simulink model "FUNCTIONING_SC"  (R2022b)
settings: Solver=FixedStepAuto  StartTime=0.0  StopTime=10.0  FixedStep=1e-3  RelTol=1e-3  EnableMultiTasking=on
undefined symbols (not defined in the file): D0, D1, D10, D11, D12, D13, D2, D3, D4, D5, D6, D7, D8, D9, PTA0, PTA1, PTA2, PTB23, PTB9, PTC16, PTC17, PTC2, PTC3, PTC4, PTD0, PTD1, PTD2, PTD3
libraries: frdmk64flib x19, etargetslib x3
settings Model: ExtModeTrigDuration=5  Creator=Hakam  LastModifiedBy=Hakam
settings OptimizationCC: EnhancedBackFolding=on  PassReuseOutputArgsAs=Individual arguments  ZeroExternalMemoryAtStartup=off  ZeroInternalMemoryAtStartup=off  MaxStackSize=64  OptimizeBlockOrder=speed  DifferentSizesBufferReuse=on  OptimizationCustomize=off  EfficientTunableParamExpr=on
settings DebuggingCC: ParameterTunabilityLossMsg=error
settings HardwareCC: ProdBitPerPointer=32  ProdBitPerSizeT=32  ProdBitPerPtrDiffT=32  ProdLargestAtomicInteger=Long  ProdLargestAtomicFloat=Double  ProdWordSize=32  ProdHWDeviceType=ARM Compatible->ARM Cortex
settings SFSimCC: MATLABDynamicMemAlloc=off
settings RTWCC: Description=Embedded Coder  SystemTargetFile=ert.tlc  HardwareBoard=NXP FRDM-K64F  TLCOptions="-aInlineSetEventsForThisBaseRateFcn=TLC_FALSE -aSuppressMultiTaskScheduler=TLC_FALSE  -aRateBasedStepFcn=0"  TemplateMakefile=ert_default_tmf  Toolchain=GNU Tools for ARM Embedded Processors
settings CodeAppCC: ForceParamTrailComments=on  IgnoreCustomStorageClasses=off  OperatorAnnotations=on  SimulinkDataObjDesc=on  SFDataObjDesc=on  InsertBlockDesc=on
settings ERTTargetCC: ExtModeTransport=4  ExtModeMexFile=sendToCommService

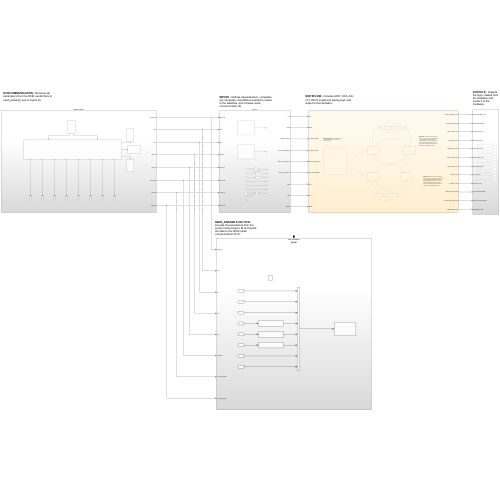
[thumbnail: Simulink's stored preview of the top-level diagram]
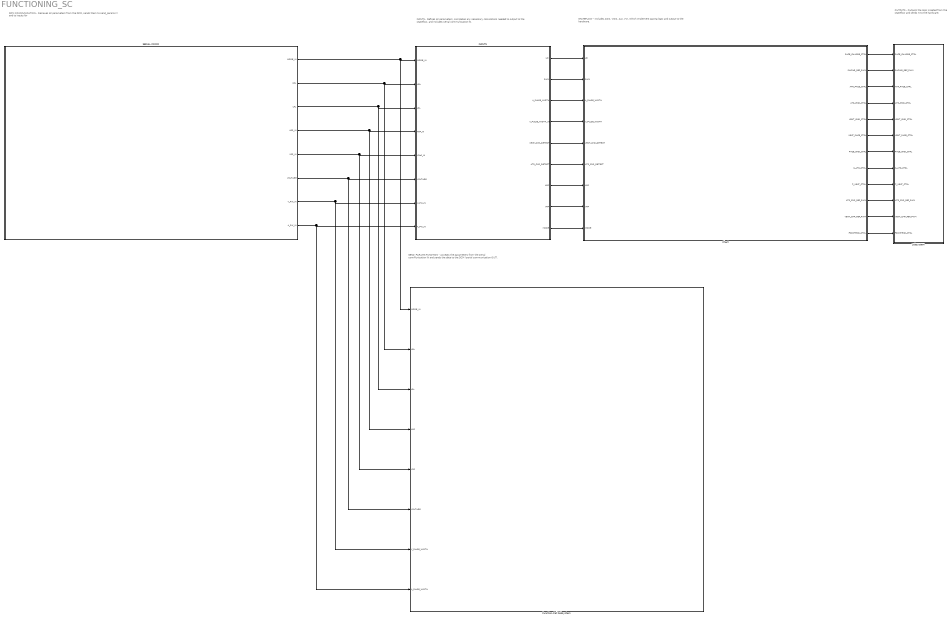
== system FUNCTIONING_SC ==
  note: INPUTS - Defines all parameters, completes any necessary calculations needed to output to the stateflow, and includes serial communication IN.
  note: STATEFLOW - Includes AOO, VOO, AAI, VVI, Which implement pacing logic and output to the hardware.
  note: SEND_PARAMS FUNCTION - Accepts the parameters from the serial communication IN and sends the data to the DCM (serial communication OUT).
  note: OUTPUTS - Outputs the logic created from the stateflow and sends it to the hardware.
  note: DCM COMMUNICATION - Recieves all parameters from the DCM, sends them to send_params() and to inputs for
  Chart : Stateflow chart  TreatAsAtomicUnit=on
      settings: PortSchema="{\"entries\":[{\"content\":{\"sides\":[{\"content\":{\"connectorIds\":[\"In5\",\"In2\",\"In1\",\"In7\",\"In3\",\"In4\",\"In6\",\"In9\",\"In8\"]},\"type\":\"ConnectorPlacement.EquallySpacedRectSide\",\"uuid\":\"579a0715-eecf-4ad1-b9c7-876da5a2f487\"},{\"content\":{\"connectorIds\":[\"Out1\",\"Out2\",\"Out3\",\"Out4\",\"Out5\",\"Out6\",\"Out7\",\"Out8\",\"Out9\",\"Out10\",\"Out11\",\"Out12\"],\"side\":\"RIGHT\"},\"type\":\"ConnectorPlacement.EquallySpacedRectSide\",\"uuid\":\"7723b8dd-9321-4ba0-a105-5fe980f58500\"},{\"content\":{\"connectorIds\":[],\"side\":\"TOP\"},\"type\":\"ConnectorPlacement.EquallySpacedRectSide\",\"uuid\":\"a2cc372f-b65a-4c95-aa24-637f5fae7d8b\"}]},\"type\":\"ConnectorPlacement.EquallySpacedConnector\",\"uuid\":\"f3293a12-0736-4187-8ed2-302834bf53da\"}],\"packageUris\":[\"http://schema.mathworks.com/mf0/Connector/R2020b\"],\"version\":\"1.0\"}"
  Function-Call Subsystem : Subsystem  TreatAsAtomicUnit=on
  INPUTS : Subsystem
      settings: PortSchema="{\"entries\":[{\"content\":{\"sides\":[{\"content\":{\"connectorIds\":[]},\"type\":\"ConnectorPlacement.EquallySpacedRectSide\",\"uuid\":\"bedbe6ad-1dc2-4cce-9585-188ab1dfdae5\"},{\"content\":{\"connectorIds\":[],\"side\":\"RIGHT\"},\"type\":\"ConnectorPlacement.EquallySpacedRectSide\",\"uuid\":\"0b0c00e6-e38b-4dbd-945a-73b1885ed563\"},{\"content\":{\"connectorIds\":[\"In1\",\"In2\",\"In3\",\"In4\",\"In5\",\"In6\",\"In7\",\"In8\"],\"side\":\"TOP\"},\"type\":\"ConnectorPlacement.EquallySpacedRectSide\",\"uuid\":\"0c1f6ce2-499b-446e-a336-8c6519be34d0\"},{\"content\":{\"connectorIds\":[\"Out1\",\"Out2\",\"Out3\",\"Out4\",\"Out5\",\"Out6\",\"Out7\",\"Out8\",\"Out9\"],\"side\":\"BOTTOM\"},\"type\":\"ConnectorPlacement.EquallySpacedRectSide\",\"uuid\":\"510989f2-1dca-4772-b500-383bd8bd4f04\"}]},\"type\":\"ConnectorPlacement.EquallySpacedConnector\",\"uuid\":\"2b867d07-0d3f-4ca3-b154-a8d01fc9a05c\"}],\"packageUris\":[\"http://schema.mathworks.com/mf0/Connector/R2020b\"],\"version\":\"1.0\"}"
  SERIAL COMM : Subsystem
      settings: PortSchema="{\"entries\":[{\"content\":{\"sides\":[{\"content\":{\"connectorIds\":[]},\"type\":\"ConnectorPlacement.EquallySpacedRectSide\",\"uuid\":\"bedbe6ad-1dc2-4cce-9585-188ab1dfdae5\"},{\"content\":{\"connectorIds\":[],\"side\":\"RIGHT\"},\"type\":\"ConnectorPlacement.EquallySpacedRectSide\",\"uuid\":\"0b0c00e6-e38b-4dbd-945a-73b1885ed563\"},{\"content\":{\"connectorIds\":[],\"side\":\"TOP\"},\"type\":\"ConnectorPlacement.EquallySpacedRectSide\",\"uuid\":\"0c1f6ce2-499b-446e-a336-8c6519be34d0\"},{\"content\":{\"connectorIds\":[\"Out1\",\"Out2\",\"Out3\",\"Out4\",\"Out5\",\"Out6\",\"Out7\",\"Out8\"],\"side\":\"BOTTOM\"},\"type\":\"ConnectorPlacement.EquallySpacedRectSide\",\"uuid\":\"510989f2-1dca-4772-b500-383bd8bd4f04\"}]},\"type\":\"ConnectorPlacement.EquallySpacedConnector\",\"uuid\":\"2b867d07-0d3f-4ca3-b154-a8d01fc9a05c\"}],\"packageUris\":[\"http://schema.mathworks.com/mf0/Connector/R2020b\"],\"version\":\"1.0\"}"
  Subsystem : Subsystem
  wires:
  SERIAL COMM/4(ARP_IN) -> Function-Call Subsystem/4(ARP), INPUTS/4(ARP_IN)
  INPUTS/6(ATR_CMP_DETECT) -> Chart/4(ATR_CMP_DETECT)
  INPUTS/2(PWM) -> Chart/2(PWM)
  INPUTS/7(ARP) -> Chart/6(ARP)
  Chart/6(VENT_PACE_CTRL) -> Subsystem/6(VENT_PACE_CTRL)
  INPUTS/9(MODE) -> Chart/8(MODE)
  INPUTS/4(V_PULSE_WIDTH_IN) -> Chart/7(V_PULSE_WIDTH)
  SERIAL COMM/7(V_PW_IN) -> INPUTS/7(V_PW_IN), Function-Call Subsystem/7(V_PULSE_WIDTH)
  INPUTS/8(VRP) -> Chart/9(VRP)
  Chart/3(ATR_PACE_CTRL) -> Subsystem/3(ATR_PACE_CTRL)
  Chart/8(Z_ATR_CTRL) -> Subsystem/8(Z_ATR_CTRL)
  Chart/9(Z_VENT_CTRL) -> Subsystem/9(Z_VENT_CTRL)
  SERIAL COMM/5(VRP_IN) -> Function-Call Subsystem/5(VRP), INPUTS/5(VRsP_IN)
  SERIAL COMM/1(MODE_IN) -> Function-Call Subsystem/1(MODE_IN), INPUTS/1(MODE_IN)
  Chart/10(ATR_CMP_REF_PWM) -> Subsystem/10(ATR_CMP_REF_PWM)
  Chart/5(VENT_GND_CTRL) -> Subsystem/5(VENT_GND_CTRL)
  Chart/12(FRONTEND_CTRL) -> Subsystem/12(FRONTEND_CTRL)
  Chart/4(ATR_GND_CTRL) -> Subsystem/4(ATR_GND_CTRL)
  Chart/7(PACE_GND_CTRL) -> Subsystem/7(PACE_GND_CTRL)
  Chart/11(VENT_CMP_REF_PWM) -> Subsystem/11(VENT_CMP_REF_PWM)
  Chart/1(PACE_CHARGE_CTRL) -> Subsystem/1(PACE_CHARGE_CTRL)
  SERIAL COMM/6(VOLTAGE) -> Function-Call Subsystem/6(VOLTAGE), INPUTS/6(VOLTAGE)
  Chart/2(PACING_REF_PWM) -> Subsystem/2(PACING_REF_PWM)
  INPUTS/5(VENT_CMP_DETECT) -> Chart/3(VENT_CMP_DETECT)
  SERIAL COMM/3(LRL) -> INPUTS/3(LRL), Function-Call Subsystem/3(LRL)
  INPUTS/1(LRI) -> Chart/5(LRI)
  INPUTS/3(A_PULSE_WIDTH) -> Chart/1(A_PULSE_WIDTH)
  SERIAL COMM/2(URL) -> INPUTS/2(URL), Function-Call Subsystem/2(URL)
  SERIAL COMM/8(A_PW_IN) -> INPUTS/8(A_PW_IN), Function-Call Subsystem/8(A_PULSE_WIDTH)

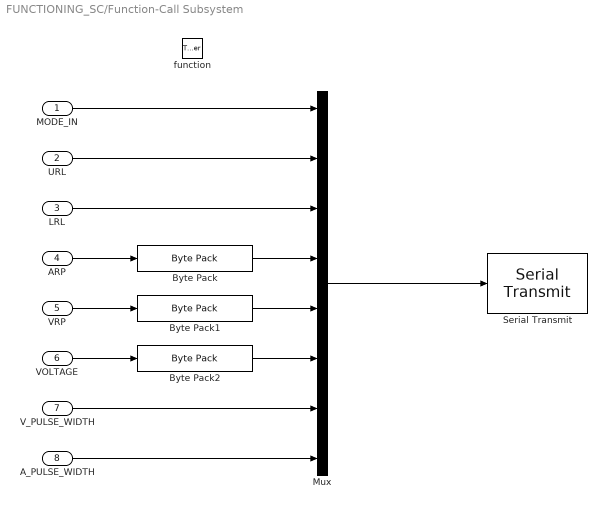
== system FUNCTIONING_SC/Function-Call Subsystem ==
  MODE_IN : Inport
  URL : Inport  Port=2
  LRL : Inport  Port=3
  ARP : Inport  Port=4
  VRP : Inport  Port=5
  VOLTAGE : Inport  Port=6  OutDataTypeStr=single
  V_PULSE_WIDTH : Inport  Port=7
  A_PULSE_WIDTH : Inport  Port=8
  function : TriggerPort  TriggerType=function-call  IsSimulinkFunction=on  FunctionName=send_parameters  VariantControl=(inherit)
  Byte Pack : etargetslib/Byte Pack  datatypes={'uint16'}  byteAlign=1
  Byte Pack1 : etargetslib/Byte Pack  datatypes={'uint16'}  byteAlign=1
  Byte Pack2 : etargetslib/Byte Pack  datatypes={'single'}  byteAlign=1
  Mux : Mux  Inputs=8
  Serial Transmit : frdmk64flib/Serial Transmit  SCIModule=0  Baudrate=uint32(9600)  Parity=None  StopBits=1  HardwareFlowControl=None  ByteOrder=LittleEndian  BlockingMode=on  OutputStatus=off
  wires:
  Mux/1 -> Serial Transmit/1
  A_PULSE_WIDTH/1 -> Mux/8
  Byte Pack/1 -> Mux/4
  ARP/1 -> Byte Pack/1
  VRP/1 -> Byte Pack1/1
  Byte Pack1/1 -> Mux/5
  V_PULSE_WIDTH/1 -> Mux/7
  MODE_IN/1 -> Mux/1
  LRL/1 -> Mux/3
  URL/1 -> Mux/2
  Byte Pack2/1 -> Mux/6
  VOLTAGE/1 -> Byte Pack2/1

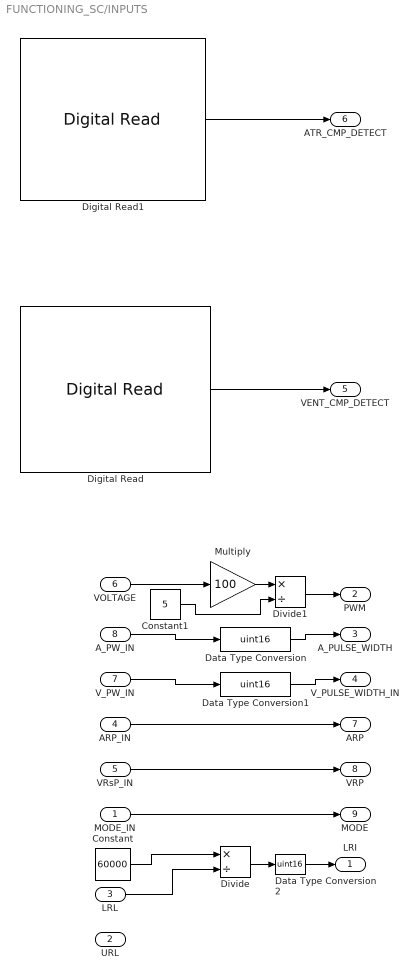
== system FUNCTIONING_SC/INPUTS ==
  MODE_IN : Inport
  URL : Inport  Port=2
  LRL : Inport  Port=3
  ARP_IN : Inport  Port=4
  VRsP_IN : Inport  Port=5
  VOLTAGE : Inport  Port=6
  V_PW_IN : Inport  Port=7
  A_PW_IN : Inport  Port=8
  Constant : Constant  Value=60000
  Constant1 : Constant  Value=5
  Data Type Conversion : DataTypeConversion  OutDataTypeStr=uint16  SaturateOnIntegerOverflow=off  RndMeth=Floor
  Data Type Conversion1 : DataTypeConversion  OutDataTypeStr=uint16  SaturateOnIntegerOverflow=off  RndMeth=Floor
  Data Type Conversion2 : DataTypeConversion  OutDataTypeStr=uint16  SaturateOnIntegerOverflow=off  RndMeth=Floor
  Digital Read : frdmk64flib/Digital Read  Whichpin=PTC17 (D1)  SampleTime=-1
  Digital Read1 : frdmk64flib/Digital Read  Whichpin=PTC16 (D0)  SampleTime=-1
  Divide : Product  Inputs=*/
  Divide1 : Product  Inputs=*/
  Multiply : Gain  Gain=100
  LRI : Outport
  PWM : Outport  Port=2
  A_PULSE_WIDTH : Outport  Port=3
  V_PULSE_WIDTH_IN : Outport  Port=4
  VENT_CMP_DETECT : Outport  Port=5
  ATR_CMP_DETECT : Outport  Port=6
  ARP : Outport  Port=7
  VRP : Outport  Port=8
  MODE : Outport  Port=9
  wires:
  Digital Read1/1 -> ATR_CMP_DETECT/1
  Digital Read/1 -> VENT_CMP_DETECT/1
  LRL/1 -> Divide/2
  Divide/1 -> Data Type Conversion2/1
  Constant1/1 -> Divide1/2
  Multiply/1 -> Divide1/1
  Divide1/1 -> PWM/1
  Data Type Conversion/1 -> A_PULSE_WIDTH/1
  Data Type Conversion1/1 -> V_PULSE_WIDTH_IN/1
  ARP_IN/1 -> ARP/1
  VRsP_IN/1 -> VRP/1
  MODE_IN/1 -> MODE/1
  Constant/1 -> Divide/1
  A_PW_IN/1 -> Data Type Conversion/1
  Data Type Conversion2/1 -> LRI/1
  VOLTAGE/1 -> Multiply/1
  V_PW_IN/1 -> Data Type Conversion1/1

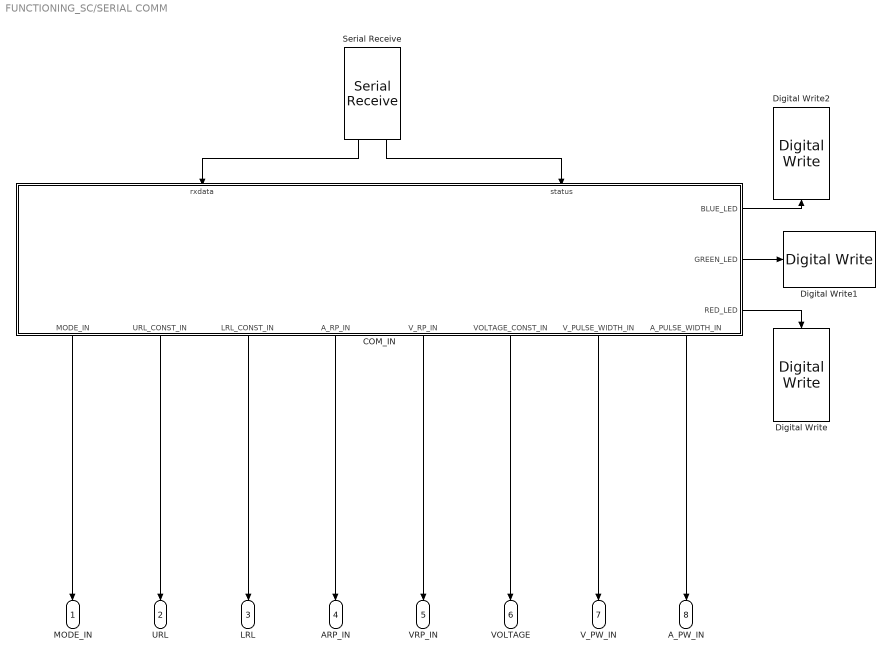
== system FUNCTIONING_SC/SERIAL COMM ==
  COM_IN : Stateflow chart  TreatAsAtomicUnit=on
      settings: PortSchema="{\"entries\":[{\"content\":{\"sides\":[{\"content\":{\"connectorIds\":[\"In1\",\"In2\"]},\"type\":\"ConnectorPlacement.EquallySpacedRectSide\",\"uuid\":\"d63df865-b51f-43d6-a13f-6ae075812ede\"},{\"content\":{\"connectorIds\":[\"Out6\",\"Out9\",\"Out4\",\"Out5\",\"Out8\",\"Out3\",\"Out7\",\"Out2\"],\"side\":\"RIGHT\"},\"type\":\"ConnectorPlacement.EquallySpacedRectSide\",\"uuid\":\"8033d1cf-b8ff-4fd5-8be7-20697f5f926f\"},{\"content\":{\"connectorIds\":[],\"side\":\"TOP\"},\"type\":\"ConnectorPlacement.EquallySpacedRectSide\",\"uuid\":\"dd3d3828-7779-4157-9ae9-dc8022e14938\"},{\"content\":{\"connectorIds\":[\"Out1\",\"Out11\",\"Out10\"],\"side\":\"BOTTOM\"},\"type\":\"ConnectorPlacement.EquallySpacedRectSide\",\"uuid\":\"0a7ca57a-2a94-44e2-b41b-d07737135386\"}]},\"type\":\"ConnectorPlacement.EquallySpacedConnector\",\"uuid\":\"07d8ed07-1da2-4ca8-9f50-15ba3dce33e0\"}],\"packageUris\":[\"http://schema.mathworks.com/mf0/Connector/R2020b\"],\"version\":\"1.0\"}"
  Digital Write : frdmk64flib/Digital Write  Whichpin=RED_LED
  Digital Write1 : frdmk64flib/Digital Write  Whichpin=GREEN_LED
  Digital Write2 : frdmk64flib/Digital Write  Whichpin=BLUE_LED
  Serial Receive : frdmk64flib/Serial Receive  SCIModule=0  Baudrate=uint32(9600)  Parity=None  StopBits=1  HardwareFlowControl=None  ByteOrder=LittleEndian  DataType=uint8  DataLength=15  BlockingMode=off  OutputStatus=on  SampleTime=-1
  MODE_IN : Outport
  URL : Outport  Port=2
  LRL : Outport  Port=3
  ARP_IN : Outport  Port=4
  VRP_IN : Outport  Port=5
  VOLTAGE : Outport  Port=6  OutDataTypeStr=single
  V_PW_IN : Outport  Port=7
  A_PW_IN : Outport  Port=8
  wires:
  COM_IN/3(VOLTAGE_CONST_IN) -> VOLTAGE/1
  Serial Receive/2 -> COM_IN/2(status)
  Serial Receive/1 -> COM_IN/1(rxdata)
  COM_IN/2(A_PULSE_WIDTH_IN) -> A_PW_IN/1
  COM_IN/5(A_RP_IN) -> ARP_IN/1
  COM_IN/6(MODE_IN) -> MODE_IN/1
  COM_IN/7(V_PULSE_WIDTH_IN) -> V_PW_IN/1
  COM_IN/8(V_RP_IN) -> VRP_IN/1
  COM_IN/4(LRL_CONST_IN) -> LRL/1
  COM_IN/9(URL_CONST_IN) -> URL/1
  COM_IN/10(RED_LED) -> Digital Write/1
  COM_IN/11(GREEN_LED) -> Digital Write1/1
  COM_IN/1(BLUE_LED) -> Digital Write2/1

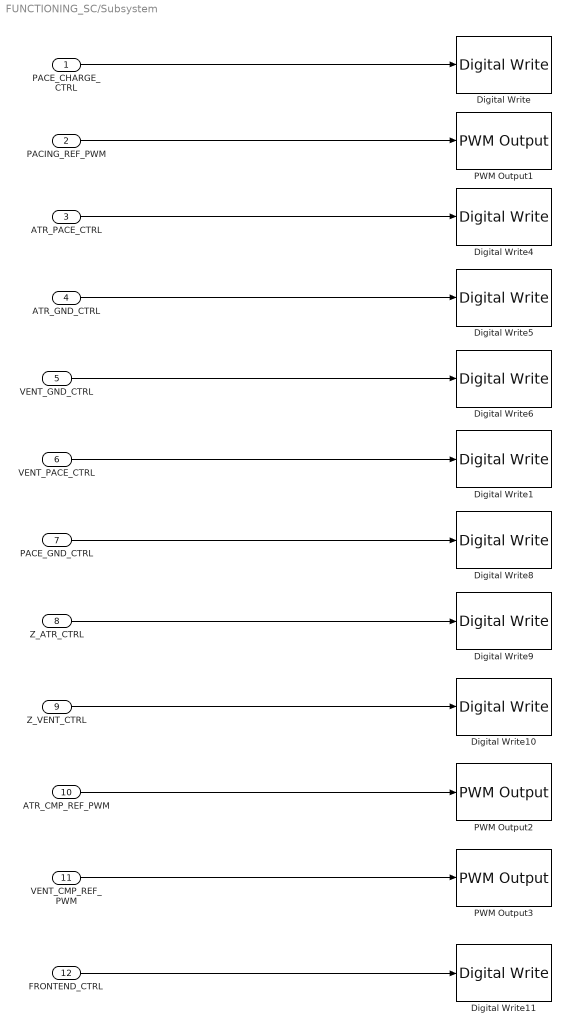
== system FUNCTIONING_SC/Subsystem ==
  PACE_CHARGE_CTRL : Inport
  PACING_REF_PWM : Inport  Port=2
  ATR_PACE_CTRL : Inport  Port=3
  ATR_GND_CTRL : Inport  Port=4
  VENT_GND_CTRL : Inport  Port=5
  VENT_PACE_CTRL : Inport  Port=6
  PACE_GND_CTRL : Inport  Port=7
  Z_ATR_CTRL : Inport  Port=8
  Z_VENT_CTRL : Inport  Port=9
  ATR_CMP_REF_PWM : Inport  Port=10
  VENT_CMP_REF_PWM : Inport  Port=11
  FRONTEND_CTRL : Inport  Port=12
  Digital Write : frdmk64flib/Digital Write  Whichpin=PTB9 (D2)
  Digital Write1 : frdmk64flib/Digital Write  Whichpin=PTC4 (D9)
  Digital Write10 : frdmk64flib/Digital Write  Whichpin=PTC3 (D7)
  Digital Write11 : frdmk64flib/Digital Write  Whichpin=PTD1 (D13)
  Digital Write4 : frdmk64flib/Digital Write  Whichpin=PTA0 (D8)
  Digital Write5 : frdmk64flib/Digital Write  Whichpin=PTD2 (D11)
  Digital Write6 : frdmk64flib/Digital Write  Whichpin=PTD3 (D12)
  Digital Write8 : frdmk64flib/Digital Write  Whichpin=PTD0 (D10)
  Digital Write9 : frdmk64flib/Digital Write  Whichpin=PTB23 (D4)
  PWM Output1 : frdmk64flib/PWM Output  Whichpin=PTA2 (D5)  InitialFrequency=2000  InitialDutyCycle=100
  PWM Output2 : frdmk64flib/PWM Output  Whichpin=PTC2 (D6)  InitialFrequency=2000  InitialDutyCycle=0
  PWM Output3 : frdmk64flib/PWM Output  Whichpin=PTA1 (D3)  InitialFrequency=2000  InitialDutyCycle=0
  wires:
  PACE_CHARGE_CTRL/1 -> Digital Write/1
  PACING_REF_PWM/1 -> PWM Output1/1
  ATR_PACE_CTRL/1 -> Digital Write4/1
  ATR_GND_CTRL/1 -> Digital Write5/1
  VENT_GND_CTRL/1 -> Digital Write6/1
  VENT_PACE_CTRL/1 -> Digital Write1/1
  PACE_GND_CTRL/1 -> Digital Write8/1
  Z_ATR_CTRL/1 -> Digital Write9/1
  Z_VENT_CTRL/1 -> Digital Write10/1
  VENT_CMP_REF_PWM/1 -> PWM Output3/1
  ATR_CMP_REF_PWM/1 -> PWM Output2/1
  FRONTEND_CTRL/1 -> Digital Write11/1

== stateflow chart FUNCTIONING_SC/SERIAL COMM/COM_IN ==
  state SET_PARAM
    entry:
    MODE_IN = rxdata(3); %Pacing modes (1-4)
    URL_CONST_IN = rxdata(4); %Upper rate limit (ppm)
    LRL_CONST_IN = rxdata(5); %Lower rate limit (ppm)
    A_RP_IN = typecast(rxdata(6:7), 'uint16'); %Refractory period (ms)
    V_RP_IN = typecast(rxdata(8:9), 'uint16'); %Refractory period (ms)
    VOLTAGE_CONST_IN =  typecast(rxdata(10:13), 'single'); %Pulse Amplitude (V)
    V_PULSE_WIDTH_IN = rxdata(14); %Pulse width (ms)
    A_PULSE_WIDTH_IN = rxdata(15); %Pulse width (ms)
    GREEN_LED=1;
    BLUE_LED = 0;
    RED_LED = 0;
  state INITIAL
    entry:
    A_PULSE_WIDTH_IN = 1;
    V_PULSE_WIDTH_IN = 2;
    VOLTAGE_CONST_IN = 1;
    LRL_CONST_IN = 1;
    A_RP_IN = 1;
    V_RP_IN = 1;
    MODE_IN = 3;
  state STANDBY
    entry:
    RED_LED=1;
    BLUE_LED = 0;
    GREEN_LED=0;
  state ECHO_PARAM
    entry:
    RED_LED = 0;
    BLUE_LED = 1;
    send_parameters();
  SET_PARAM -> STANDBY : [after(500,msec)]
  (default) -> INITIAL
  (junction 15) -> SET_PARAM [order 1] : [rxdata(2)==hex2dec('55')]
  (junction 14) -> STANDBY [order 2]
  INITIAL -> STANDBY
  STANDBY -> (junction 14) : [status==0]
  (junction 14) -> (junction 15) [order 1] : [rxdata(1)==hex2dec('16')]
  (junction 15) -> ECHO_PARAM [order 2] : [rxdata(2)==hex2dec('22')]
  ECHO_PARAM -> STANDBY : [after(500,msec)]
  data: BLUE_LED output; rxdata input uint8; A_PULSE_WIDTH_IN output uint8; VOLTAGE_CONST_IN output single; LRL_CONST_IN output uint8; A_RP_IN output uint16; MODE_IN output uint8; V_PULSE_WIDTH_IN output uint8; V_RP_IN output uint16; URL_CONST_IN output uint8; status input uint8; RED_LED output; GREEN_LED output

== stateflow chart FUNCTIONING_SC/Chart ==
  state ARP
    entry:
    FRONTEND_CTRL=true;
  state ALERT_A
    entry:
    FRONTEND_CTRL=true;
  note: AOO/AAI - Performs the pacing for the atrium. for AOO, the heart will be paced regardless of the heart's natural behaviour, while for AAI the heat will be paced based on the lower rate limit IF the natural heart behaviour is unalligned with it.
  note: INITIALIZATION - Initialzes all the pins that are to be used in the pacing modes.
  state DISCHARGE_CHARGE_A
    entry:
    PACE_CHARGE_CTRL=true;
    PACE_GND_CTRL=true;
    VENT_PACE_CTRL=false;
    ATR_PACE_CTRL=false;
    VENT_GND_CTRL=false;
    ATR_GND_CTRL=true;
  state PACE_A
    entry:
    PACE_CHARGE_CTRL=false;
    VENT_GND_CTRL=false;
    ATR_GND_CTRL=false;
    PACE_GND_CTRL=true;
    VENT_PACE_CTRL=false;
    ATR_PACE_CTRL=true;
  state INIT
    entry:
    PACING_REF_PWM=PWM;
    PACE_CHARGE_CTRL=false;
    VENT_PACE_CTRL=false;
    ATR_PACE_CTRL=false;
    VENT_GND_CTRL=false;
    ATR_GND_CTRL=false;
    PACE_GND_CTRL=false;
    Z_ATR_CTRL=false;
    Z_VENT_CTRL=false;
    FRONTEND_CTRL=true;
    VENT_CMP_REF_PWM=90;
    ATR_CMP_REF_PWM=90;
  state DISCHARGE_CHARGE_V
    entry:
    PACE_CHARGE_CTRL=true;
    PACE_GND_CTRL=true;
    VENT_PACE_CTRL=false;
    ATR_PACE_CTRL=false;
    VENT_GND_CTRL=true;
    ATR_GND_CTRL=false;
  state PACE_V
    entry:
    PACE_CHARGE_CTRL=false;
    VENT_GND_CTRL=false;
    ATR_GND_CTRL=false;
    PACE_GND_CTRL=true;
    VENT_PACE_CTRL=true;
    ATR_PACE_CTRL=false;
  note: VOO/VVI - Performs the pacing for the ventricle. for VOO, the heart will be paced regardless of the heart's natural behaviour, while for VVI the heat will be paced based on the lower rate limit IF the natural heart behaviour is unalligned with it.
  state VRP
    entry:
    FRONTEND_CTRL=true;
  state ALERT_V
    entry:
    FRONTEND_CTRL=true;
  ALERT_A -> ARP [order 1] : [ATR_CMP_DETECT==true]
  DISCHARGE_CHARGE_A -> ARP [order 2] : [MODE==3]
  ALERT_A -> PACE_A [order 2] : [after(LRI-ARP,msec)]
  ARP -> ALERT_A : [after(ARP-A_PULSE_WIDTH,msec)]
  DISCHARGE_CHARGE_A -> PACE_A [order 1] : [after(LRI-A_PULSE_WIDTH,msec) && MODE==1 ]
  (default) -> INIT
  INIT -> DISCHARGE_CHARGE_A [order 1] : [MODE==1 | MODE == 3]
  PACE_A -> DISCHARGE_CHARGE_A : [after(A_PULSE_WIDTH,msec)]
  DISCHARGE_CHARGE_V -> PACE_V [order 1] : [after(LRI-V_PULSE_WIDTH,msec) && MODE==2]
  INIT -> DISCHARGE_CHARGE_V [order 2] : [MODE==2 | MODE==4]
  DISCHARGE_CHARGE_V -> VRP [order 2] : [MODE==4]
  PACE_V -> DISCHARGE_CHARGE_V : [after(V_PULSE_WIDTH,msec)]
  ALERT_V -> PACE_V [order 2] : [after(LRI-VRP,msec)]
  ALERT_V -> VRP [order 1] : [VENT_CMP_DETECT==true]
  VRP -> ALERT_V : [after(VRP-V_PULSE_WIDTH,msec)]
  data: A_PULSE_WIDTH input; PACE_CHARGE_CTRL output; PACING_REF_PWM output double; ATR_PACE_CTRL output; ATR_GND_CTRL output; VENT_GND_CTRL output; VENT_PACE_CTRL output; PACE_GND_CTRL output; Z_ATR_CTRL output; Z_VENT_CTRL output; PWM input double; VENT_CMP_DETECT input; ATR_CMP_DETECT input; LRI input; ARP input; V_PULSE_WIDTH input; MODE input; ATR_CMP_REF_PWM output; VENT_CMP_REF_PWM output; FRONTEND_CTRL output; VRP input
